simulink model "Inductive_Load_PID"  (R2021a)
settings: Solver=VariableStepAuto  StartTime=0.0  StopTime=0.2  RelTol=1e-3  AbsTol=1e-3  EnableMultiTasking=on
StopFcn:
  | ee_addSimlogTimeStamp(bdroot)
libraries: fl_lib x10, ee_lib x7, nesl_utility x7, simulink x1, pid_lib x1, spsTriangleGeneratorLib x1
CloseFcn:
  | try,close(h1_ee_motor_dc_pwm),end
  | clear h1_ee_motor_dc_pwm
  | 
  | clear simlog_ee_motor_dc_pwm
  | clear logsout_ee_motor_dc_pwm
  | clear RPM RPM1 tout
Description:
  | PWM-Controlled DC Motor
settings Model: Creator=The MathWorks, Inc.  LastModifiedBy=PHsco
settings SolverCC: AutoScaleAbsTol=off
settings DataIOCC: LimitDataPoints=on  MaxDataPoints=10000  SaveFormat=Array  ReturnWorkspaceOutputs=off  SignalLoggingName=logsout_ee_motor_dc_pwm
settings OptimizationCC: ExpressionDepthLimit=2147483647  InitFltsAndDblsToZero=on  LifeSpan=inf
settings DebuggingCC: UnderspecifiedInitializationDetection=Classic  MergeDetectMultiDrivingBlocksExec=none  FcnCallInpInsideContextMsg=warning  StateNameClashWarn=warning  SFUnexpectedBacktrackingDiag=warning  SFNoUnconditionalDefaultTransitionDiag=warning  SFExecutionAtInitializationDiag=none  SFMachineParentedDataDiag=warning  ArithmeticOperatorsInVariantConditions=warning
settings HardwareCC: ProdBitPerPointer=32  ProdBitPerSizeT=32  ProdBitPerPtrDiffT=32  ProdLargestAtomicFloat=None  ProdIntDivRoundTo=Undefined  ProdEndianess=Unspecified  ProdWordSize=32  ProdHWDeviceType=32-bit Generic
settings ModelReferenceCC: PropagateSignalLabelsOutOfModel=off
settings SFSimCC: SimUseLocalCustomCode=off  CustomCodeUndefinedFunction=UseInterfaceOnly
settings RTWCC: RTWUseLocalCustomCode=off
settings CodeAppCC: StateflowObjectComments=on
settings GRTTargetCC: TargetLangStandard=C89/C90 (ANSI)  CombineOutputUpdateFcns=off  GRTInterface=on
settings ConfigComp: CovMetricSettings=dw  CovSaveCumulativeToWorkspaceVar=on  CovSaveSingleToWorkspaceVar=on  CovExternalEMLEnable=off  CovSFcnEnable=off
settings SimscapeCC: SimscapeLogType=all  SimscapeLogSimulationStatistics=on  SimscapeLogName=simlog_ee_motor_dc_pwm  SimscapeLogDataHistory=10000

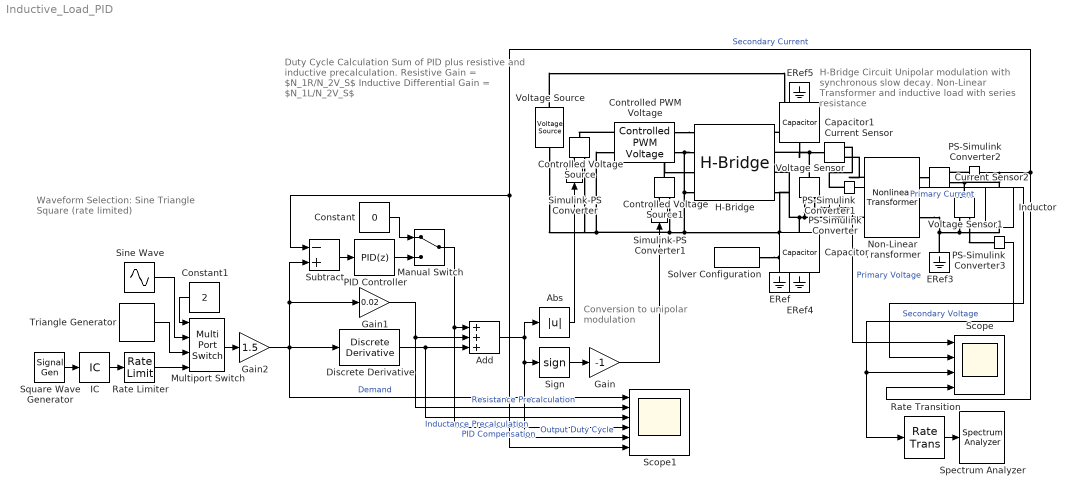
== system Inductive_Load_PID ==
  note: Duty Cycle Calculation
      | Sum of PID plus resistive and inductive precalculation.
      | Resistive Gain = $N_1R/N_2V_S$
      | Inductive Differential Gain = $N_1L/N_2V_S$
  note: Conversion to unipolar modulation
  note: Waveform Selection:
      | Sine
      | Triangle
      | Square (rate limited)
  note: H-Bridge Circuit
      | Unipolar modulation with synchronous slow decay.
      | Non-Linear Transformer and inductive load with series resistance
  Abs : Abs
  Add : Sum  Inputs=+++
  Capacitor : ee_lib/Passive/Capacitor  cap_option=0  c=10 nF  Cvec=[1e-05, 1e-06] F  Vvec=[0, 10] V  CV_table_symmetry=1  f_vec=[1, 10] kHz  DFext_vec=[.8, 1.2]  C_tol=5  enable_C_tol=0  tol_distribution=1  nSigma=4  r=1e-6 Ohm  g=0 1/Ohm  averaging_period=0 s  enable_operating_limits=0  operating_limit_action=2  max_working_voltage_range=[-25, 25] V  power_rating=1 W  enable_faults=0  fault_action=1  Cscale_faulted=100  R_faulted=1e-3 Ohm  G_faulted=0 1/Ohm  tau_fault=1e-3 s  enable_temporal_fault=0  t_fault=1 s  enable_behavioral_fault=0  max_permissible_voltage_range=[-100, 100] V  t_fail_on_voltage=1 s  i_specify=off  i_priority=None  i=0 A  i_nominal_specify=off  i_nominal_unit=A  i_nominal_value=1  v_specify=off  v_priority=None  v=0 V  v_nominal_specify=off  v_nominal_unit=V  v_nominal_value=1  vc_specify=off  vc_priority=High  vc=0 V  vc_nominal_specify=off  vc_nominal_unit=V  vc_nominal_value=1
  Capacitor1 : ee_lib/Passive/Capacitor  cap_option=0  c=10 nF  Cvec=[1e-05, 1e-06] F  Vvec=[0, 10] V  CV_table_symmetry=1  f_vec=[1, 10] kHz  DFext_vec=[.8, 1.2]  C_tol=5  enable_C_tol=0  tol_distribution=1  nSigma=4  r=1e-6 Ohm  g=0 1/Ohm  averaging_period=0 s  enable_operating_limits=0  operating_limit_action=2  max_working_voltage_range=[-25, 25] V  power_rating=1 W  enable_faults=0  fault_action=1  Cscale_faulted=100  R_faulted=1e-3 Ohm  G_faulted=0 1/Ohm  tau_fault=1e-3 s  enable_temporal_fault=0  t_fault=1 s  enable_behavioral_fault=0  max_permissible_voltage_range=[-100, 100] V  t_fail_on_voltage=1 s  i_specify=off  i_priority=None  i=0 A  i_nominal_specify=off  i_nominal_unit=A  i_nominal_value=1  v_specify=off  v_priority=None  v=0 V  v_nominal_specify=off  v_nominal_unit=V  v_nominal_value=1  vc_specify=off  vc_priority=High  vc=0 V  vc_nominal_specify=off  vc_nominal_unit=V  vc_nominal_value=1
  Constant : Constant  Value=0
  Constant1 : Constant  Value=2
  Controlled PWM Voltage : ee_lib/Integrated Circuits/Controlled PWM Voltage  F=20 kHz  TD=0 s  pulse_width_offset=0 s  pulse_min=60 ns  Vmin=0 V  Vmax=1 V  Vm=5 V  pwm_or_av=1  event_type=1  sample_time=5e-6 s  u_min=0  u_max=1
  Controlled Voltage Source : fl_lib/Electrical/Electrical Sources/Controlled Voltage Source
  Controlled Voltage Source1 : fl_lib/Electrical/Electrical Sources/Controlled Voltage Source
  Current Sensor : fl_lib/Electrical/Electrical Sensors/Current Sensor
  Current Sensor2 : fl_lib/Electrical/Electrical Sensors/Current Sensor
  Discrete Derivative : simulink/Discrete/Discrete Derivative  gainval=0.02  ICPrevScaledInput=0.0  OutMin=[]  OutMax=[]  OutDataType=fixdt(1, 16)  OutScaling=2^-10  DoSatur=off
  ERef{,3..5} (4 alike) : fl_lib/Electrical/Electrical Elements/Electrical Reference
  Gain : Gain  Gain=-1
  Gain1 : Gain  Gain=0.02
  Gain2 : Gain  Gain=1.5
  H-Bridge : ee_lib/Semiconductors & Converters/Converters/H-Bridge  supply_ports=ee.enum.supply_ports.showsupply  Venable=2.5 V  Vmax=5 V  Vreverse=0.5 V  Vbrake=2.5 V  Vm=12 V  pwm_or_av=ee.enum.pwm_or_av.pwm  regenerative_braking_mode=ee.enum.converters.regenerative_braking_mode.always_enabled  discontinuous=ee.enum.current_profile.continuous  freewheeling_mode=ee.enum.converters.freewheeling_mode.two_switches_one_diode  Ron=0.014 Ohm  Don=0.014 Ohm  Goff=1e-6 S  Rload=3.38+0.1 Ohm  Lload=1e-5 H  F=4 kHz  thermal_mass=100 J/K  initial_temperature=298.15 K  Ron2=0.1 Ohm  Don2=0.05 Ohm  Tmeas=298.15 K  Tmeas2=398.15 K
      settings: InternalSimscapePortConfiguration="{\"Bottom\":[],\"Left\":[{\"id\":\"ENA\",\"label\":\"PWM\",\"type\":\"foundation.electrical.electrical\"},{\"id\":\"REF\",\"label\":\"REF\",\"type\":\"foundation.electrical.electrical\"},{\"id\":\"REV\",\"label\":\"REV\",\"type\":\"foundation.electrical.electrical\"},{\"id\":\"BRK\",\"label\":\"BRK\",\"type\":\"foundation.electrical.electrical\"}],\"Right\":[{\"id\":\"p1\",\"label\":\"V+\",\"type\":\"foundation.electrical.electrical\"},{\"id\":\"p2\",\"label\":\"+\",\"type\":\"foundation.electrical.electrical\"},{\"id\":\"n2\",\"label\":\"-\",\"type\":\"foundation.electrical.electrical\"},{\"id\":\"n1\",\"label\":\"V-\",\"type\":\"foundation.electrical.electrical\"}],\"Top\":[]}"
  IC : InitialCondition  Value=0
  Inductor : ee_lib/Passive/Inductor  l=1e-3 H  L_tol=20  enable_L_tol=0  tol_distribution=1  nSigma=4  r=1e-3 Ohm  g=1e-12 1/Ohm  enable_operating_limits=0  operating_limit_action=2  max_working_current=1 A  power_rating=1 W  enable_faults=0  fault_action=1  lambdaPercent=50  k_faulted=0.9999  turnsShort=0  openCct=0  groundShort=0  groundShortG=0 1/Ohm  tau_fault=1e-3 s  enable_temporal_fault=0  t_fault=1 s  enable_behavioral_fault=0  max_permissible_voltage=100 V  n_fail_on_voltage=1  max_permissible_current=1 A  t_fail_on_current=1 s  i_L_specify=off  i_L_priority=High  i_L=0 A  i_L_nominal_specify=off  i_L_nominal_unit=A  i_L_nominal_value=1
  Manual Switch : ManualSwitch
  Multiport Switch : MultiPortSwitch
  Non-Linear Transformer : ee_lib/Passive/Transformers/Nonlinear Transformer  Nw=1200  Nw2=3  winding_param_option=2  Req=0.01 Ohm  Leq=0.0001 H  R_1=25.446 Ohm  L_1=220.6 mH  R_2=0 Ohm  L_2=0.7 uH  R_m=100 Ohm  parameterization_option=4  H_data=[0, 50, 100, 150, 200, 250, 300, 350, 400, 450, 500] A/m  B_data="[0, 1.4, 1.64, 1.68, 1.71, 1.73, 1.75, 1.77, 1.78, 1.79, 1.8]   T"  length_effective=0.22 m  area_effective=0.0013 m^2  L=5 H  L_sat=1e-2 H  current_data=[0, .4, .8, 1.2, 1.6, 2] A  magnetic_flux_data=[0, .161, .25, .284, .295, .299] .* 1e-3 Wb  magnetic_flux_sat=1.6e-04 Wb  dBdH0=0.04 m*T/A  B1=1.8 T  H1=500 A/m  c=0.1  K=200 A/m  alpha=1e-4  Leq_i0=0 A  L1_i0=0 A  L2_i0=0 A  x0_option=1  i_L0=0 A  phi0=0 Wb  B0=0 T  H0=0 A/m  Leq_g=1e-9 1/Ohm  L1_g=1e-9 1/Ohm  L2_g=1e-9 1/Ohm  interpolation_option=2  averaging_period=0 s
      settings: SourceProductBaseCode=PS  InternalSimscapePortConfiguration="{\"Bottom\":[],\"Left\":[{\"id\":\"p1\",\"label\":\"1+\",\"type\":\"foundation.electrical.electrical\"},{\"id\":\"n1\",\"label\":\"1-\",\"type\":\"foundation.electrical.electrical\"}],\"Right\":[{\"id\":\"p2\",\"label\":\"2+\",\"type\":\"foundation.electrical.electrical\"},{\"id\":\"n2\",\"label\":\"2-\",\"type\":\"foundation.electrical.electrical\"}],\"Top\":[]}"
  PID Controller : pid_lib/PID Controller  Controller=PID  Form=Parallel  TimeDomain=Discrete-time  UseExternalTs=off  SampleTime=0.0001  IntegratorMethod=Forward Euler  FilterMethod=Forward Euler  ControllerParametersSource=internal  P=5  I=0.1  D=0.001  UseFilter=on  N=100  TunerSelectOption=Transfer Function Based (PID Tuner App)  InitialConditionSource=internal  InitialConditionForIntegrator=0  InitialConditionForFilter=0  DifferentiatorICPrevScaledInput=0  ExternalReset=none  TrackingMode=off  Kt=1  LimitOutput=off  SatLimitsSource=internal  UpperSaturationLimit=inf  LowerSaturationLimit=-inf  LinearizeAsGain=on  AntiWindupMode=none  Kb=1  POutMin=[]  POutMax=[]  IOutMin=[]  IOutMax=[]  DOutMin=[]  DOutMax=[]  NOutMin=[]  NOutMax=[]  SumOutMin=[]  SumOutMax=[]  SaturationOutMin=[]  SaturationOutMax=[]  PParamMin=[]  PParamMax=[]  IParamMin=[]  IParamMax=[]  DParamMin=[]  DParamMax=[]  NParamMin=[]  NParamMax=[]  KbParamMin=[]  KbParamMax=[]  KtParamMin=[]  KtParamMax=[]  KbOutMin=[]  KbOutMax=[]  KtOutMin=[]  KtOutMax=[]  IntegratorOutMin=[]  IntegratorOutMax=[]  FilterOutMin=[]  FilterOutMax=[]  SumI1OutMin=[]  SumI1OutMax=[]  SumI2OutMin=[]  SumI2OutMax=[]  SumI3OutMin=[]  SumI3OutMax=[]  SumI4OutMin=[]  SumI4OutMax=[]  SumDOutMin=[]  SumDOutMax=[]  DifferentiatorOutMin=[]  DifferentiatorOutMax=[]  FilterDiffOutCoefMin=[]  FilterDiffOutCoefMax=[]  ReciprocalOutMin=[]  ReciprocalOutMax=[]  SumDenOutMin=[]  SumDenOutMax=[]  SumNumOutMin=[]  SumNumOutMax=[]  DivideOutMin=[]  DivideOutMax=[]  UdiffTsProdOutMin=[]  UdiffTsProdOutMax=[]  NTsProdOutMin=[]  NTsProdOutMax=[]  UintegralTsProdOutMin=[]  UintegralTsProdOutMax=[]  UngainTsProdOutMin=[]  UngainTsProdOutMax=[]  IntegratorContinuousStateAttributes=''  IntegratorStateMustResolveToSignalObject=off  IntegratorRTWStateStorageClass=Auto  FilterContinuousStateAttributes=''  FilterStateMustResolveToSignalObject=off  FilterRTWStateStorageClass=Auto  ParallelPVariant=InternalParameters  IdealPVariant=Disabled  IVariant=InternalParameters  DVariant=InternalParameters  IntegratorVariant=Discrete  SatVariant=Disabled  AWVariant=Passthrough  PCopyVariant=Disabled  TRVariant=Disabled  FdbkBlocksVariant=Forward  IdealPFdbkVariant=Disabled  SatFdbkVariant=Disabled  DerivativeFilterVariant=ForwardEulerFilter  NVariant=InternalParameters  NCopyVariant=Disabled  FilterICVariant=InternalICsFilter  IntegratorICVariant=InternalICs  ExternalResetVariant=Disabled  TRSumVariant=Passthrough  SumFdbkVariant=Disabled  SumVariant=Sum_PID  TsampFilterVariant=InternalTs  TsampNgainVariant=Passthrough  TsampIntegralVariant=Passthrough  ExternalSaturationOutDataTypeStr=Inherit: Same as second input
  PS-Simulink Converter{,1..3} (4 alike) : nesl_utility/PS-Simulink Converter  PhysicalDomain=network_engine_domain  SubClassName=ps_output  LeftPortType=input  RightPortType=output  PseudoPeriodic=off  Frequencies=[]  Unit=inherit  AffineConversion=off
      settings: SourceProductBaseCode=PW,SS
  Rate Limiter : RateLimiter  RisingSlewLimit=30  FallingSlewLimit=-30  SampleTimeMode=inherited
  Rate Transition : RateTransition  OutPortSampleTime=1e-5
  Scope : Scope  NumInputPorts=4
  Scope1 : Scope  NumInputPorts=6
  Sign : Signum
  Simulink-PS Converter : nesl_utility/Simulink-PS Converter  PhysicalDomain=network_engine_domain  SubClassName=ps_input  LeftPortType=input  RightPortType=output  PseudoPeriodic=off  Frequencies=[]  NoiseDistribution=none  NoiseParameters=[]  Unit=1  AffineConversion=off  FilteringAndDerivatives=provide  SimscapeFilterOrder=1  InputFilterTimeConstant=0.001  UdotUserProvided=0
      settings: SourceProductBaseCode=PW,SS
  Simulink-PS Converter1 : nesl_utility/Simulink-PS Converter  PhysicalDomain=network_engine_domain  SubClassName=ps_input  LeftPortType=input  RightPortType=output  PseudoPeriodic=off  Frequencies=[]  NoiseDistribution=none  NoiseParameters=[]  Unit=1  AffineConversion=off  FilteringAndDerivatives=provide  SimscapeFilterOrder=1  InputFilterTimeConstant=0.001  UdotUserProvided=0
      settings: SourceProductBaseCode=PW,SS
  Sine Wave : Sin  Frequency=3*2*pi  SampleTime=0
  Solver Configuration : nesl_utility/Solver Configuration  PhysicalDomain=network_engine_domain  SubClassName=solver  LeftPortType=input  RightPortType=generic  Tones=[]  Harmonics=[]  SimulateNoise=off  Profile=off  UseLocalSampling=off  EnableSwitchedLinearOptims=on  FrequencyDomain=off  UseCCode=off  RelTol=0.001  AbsTol=1e-06  MinStep=1e-09  ToWorkspace=off  RevertToSquareIcSolve=off  NumHomotopyIterations=100  PhasorMode=off  PhasorModeNumHarmonics=1  DoDC=off  ResidualTolerance=1e-9  UseLocalSolver=off  LocalSolverChoice=NE_BACKWARD_EULER_ADVANCER  LocalSolverSampleTime=5e-6  DoFixedCost=off  MaxNonlinIter=4  MaxModeIter=2  ComputeImpulses=off  ImpulseIterations=2  LinearAlgebra=auto  EquationFormulation=NE_TIME_EF  DelaysMemoryBudget=1024  AutomaticFiltering=on  FilteringTimeConstant=0.001  PartitionStorageMethod=AS_NEEDED  PartitionMemoryBudget=1024  PartitionMethod=FAST
      settings: SourceProductBaseCode=PW,SS
  Spectrum Analyzer : SpectrumAnalyzer
  Square Wave Generator : SignalGenerator  WaveForm=square  Frequency=2
  Subtract : Sum  Inputs=-+
  Triangle Generator : spsTriangleGeneratorLib/Triangle Generator  Freq=5  Phase=90  Ts=0
  Voltage Sensor : fl_lib/Electrical/Electrical Sensors/Voltage Sensor
  Voltage Sensor1 : fl_lib/Electrical/Electrical Sensors/Voltage Sensor
  Voltage Source : ee_lib/Sources/Voltage Source  dc_voltage=25 V  ac_voltage=0 V  ac_shift=0 rad  ac_frequency=60 Hz  noise_mode=0  PSD=0 V^2/Hz  repeatability=1  auto_seed=3096051531  user_seed=0  sample_time=1e-3 s  i_specify=off  i_priority=None  i=0 A  i_nominal_specify=off  i_nominal_unit=A  i_nominal_value=1  v_specify=off  v_priority=None  v=0 V  v_nominal_specify=off  v_nominal_unit=V  v_nominal_value=1
  wires:
  Abs/1 -> Simulink-PS Converter/1
  Sign/1 -> Gain/1
  Gain/1 -> Simulink-PS Converter1/1
  PS-Simulink Converter/1 -> Scope/1  "Primary Voltage"
  PS-Simulink Converter1/1 -> Scope/2  "Primary Current"
  Add/1 -> Abs/1, Scope1/5, Sign/1  "Output Duty Cycle"
  PS-Simulink Converter3/1 -> Rate Transition/1, Scope/3  "Secondary Voltage"
  PS-Simulink Converter2/1 -> Scope1/6, Subtract/1, Scope/4  "Secondary Current"
  Gain2/1 -> Subtract/2, Gain1/1, Discrete Derivative/1, Scope1/1  "Demand"
  Subtract/1 -> PID Controller/1
  Discrete Derivative/1 -> Scope1/3, Add/3  "Inductance Precalculation"
  Square Wave Generator/1 -> IC/1
  IC/1 -> Rate Limiter/1
  Manual Switch/1 -> Scope1/4, Add/1  "PID Compensation"
  Rate Transition/1 -> Spectrum Analyzer/1
  Gain1/1 -> Scope1/2, Add/2  "Resistance Precalculation"
  PID Controller/1 -> Manual Switch/2
  Constant/1 -> Manual Switch/1
  Multiport Switch/1 -> Gain2/1
  Constant1/1 -> Multiport Switch/1
  Sine Wave/1 -> Multiport Switch/2
  Triangle Generator/1 -> Multiport Switch/3
  Rate Limiter/1 -> Multiport Switch/4
  connections:
  Controlled PWM Voltage/LConn1 -- Controlled Voltage Source/LConn1
  Controlled Voltage Source1/RConn2 -- H-Bridge/RConn4 -- ERef/LConn1 -- Solver Configuration/RConn1 -- Controlled PWM Voltage/RConn2 -- H-Bridge/LConn2 -- H-Bridge/LConn4 -- Controlled Voltage Source/RConn2 -- Voltage Source/RConn1 -- Controlled PWM Voltage/LConn2
  Simulink-PS Converter/RConn1 -- Controlled Voltage Source/RConn1
  Voltage Sensor/LConn1 -- Capacitor1/LConn1 -- H-Bridge/RConn2 -- Current Sensor/LConn1
  Voltage Sensor/RConn2 -- Non-Linear Transformer/LConn2 -- Capacitor/LConn1 -- H-Bridge/RConn3
  Controlled PWM Voltage/RConn1 -- H-Bridge/LConn1
  Controlled Voltage Source1/LConn1 -- H-Bridge/LConn3
  Simulink-PS Converter1/RConn1 -- Controlled Voltage Source1/RConn1
  Non-Linear Transformer/LConn1 -- Current Sensor/RConn2
  ERef3/LConn1 -- Non-Linear Transformer/RConn2 -- Voltage Sensor1/RConn2 -- Inductor/RConn1
  Non-Linear Transformer/RConn1 -- Current Sensor2/LConn1
  Current Sensor2/RConn2 -- Inductor/LConn1 -- Voltage Sensor1/LConn1
  ERef4/LConn1 -- Capacitor/RConn1
  ERef5/LConn1 -- Capacitor1/RConn1
  Voltage Sensor/RConn1 -- PS-Simulink Converter/LConn1
  PS-Simulink Converter1/LConn1 -- Current Sensor/RConn1
  PS-Simulink Converter2/LConn1 -- Current Sensor2/RConn1
  Voltage Sensor1/RConn1 -- PS-Simulink Converter3/LConn1
  Voltage Source/LConn1 -- H-Bridge/RConn1
